simulink model "Session_3"  (R2020b)
settings: Solver=VariableStepAuto  StartTime=0.0  StopTime=inf  RelTol=1e-3
InitFcn:
  | run('Session3.m')
values from neighbouring files (symbols this model uses):
  alpha = 0.2    [Session3.m]
  D1 = randi([0,M-1 ],1,N)    [Session3.m]
  frame = [f22 f11]    [Session3.m]
  header = (-1).^H    [Session3.m]
  hh = numel(H)    [Session3.m]
  L = length(frame)    [Session3.m]
  N = 1e3    (= 1000)    [Session3.m]
  pp = 20    [Session3.m]
  Rs = 1e4    (= 10000)    [Session3.m]
  Span = 10    [Session3.m]
  SPS = 8    [Session3.m]
  stdD = std(D2)    [Session3.m]
undefined symbols (not defined in the file or in its folder): magnitude
libraries: commdigbbndam3 x7, simulink x6, commdigbbndpm3 x6, commfilt2 x2, commchan3 x1, commsink2 x1, dspstat3 x1, dspsrcs4 x1
settings Model: Creator=ali hosseini  LastModifiedBy=ali hosseini

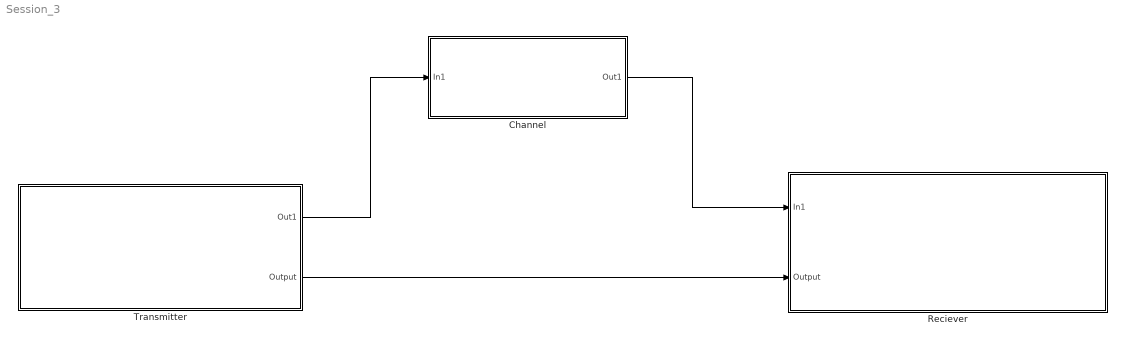
== system Session_3 ==
  Channel : Subsystem
  Reciever : Subsystem
  "Transmitter " : Subsystem
  wires:
  "Transmitter "/2(Output) -> Reciever/2(Output)
  "Transmitter "/1(Out1) -> Channel/1(In1)
  Channel/1(Out1) -> Reciever/1(In1)

== system Session_3/Channel ==
  In1 : Inport
  AWGN Channel : commchan3/AWGN Channel  InputProcessing=Columns as channels (frame based)  seed=67  noiseMode="Signal to noise ratio  (SNR)"  EbNodB=10  EsNodB=10  SNRdB=10000  bitsPerSym=1  Ps=1/SPS  Tsym=1/Rs  variance=1
  Gain : Gain  Gain=0.8
  Out1 : Outport
  wires:
  In1/1 -> AWGN Channel/1
  AWGN Channel/1 -> Gain/1
  Gain/1 -> Out1/1

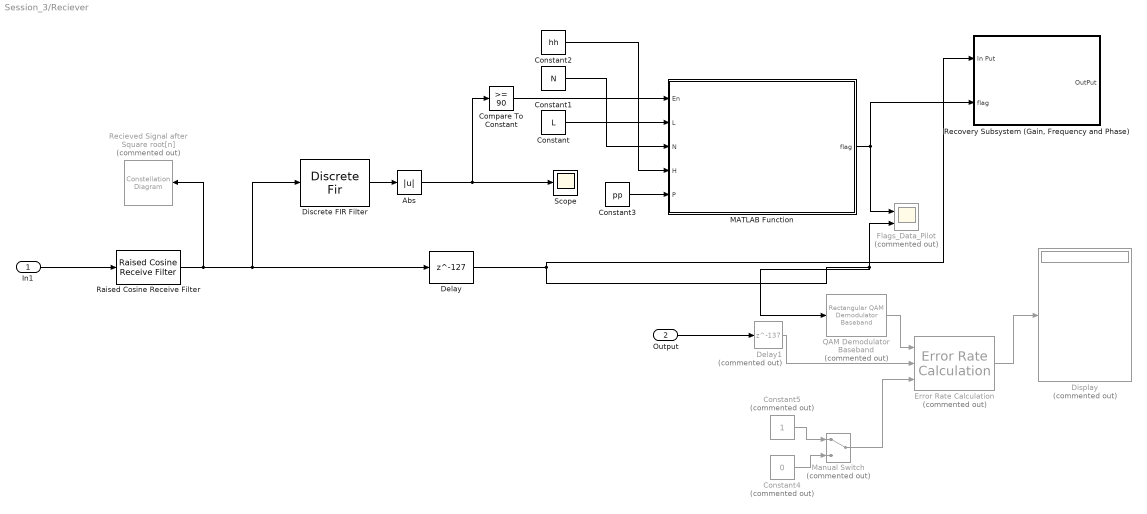
== system Session_3/Reciever ==
  In1 : Inport
  Output : Inport  Port=2
  " QAM Demodulator Baseband" : commdigbbndam3/Rectangular QAM Demodulator Baseband  Commented=on  M=M  OutType=Integer  DecType=Hard decision  VarSource=Dialog  Variance=1  Dec=Gray  Mapping=[0:15]  PowType=Min. distance between symbols  MinDist=2/stdD  AvgPow=1  PeakPow=1  Ph=0  outDtype1=Inherit via internal rule  outDtype2=Inherit via internal rule  derotateFactorWordLen=16  derotateFactorDataTypeStr=Inherit: Same word length as input  derotateFactorLastDataTypeStr=Inherit: Same word length as input  denormFactorWordLen=16  denormFactorDataTypeStr=Inherit: Same word length as input  denormFactorLastDataTypeStr=Inherit: Same word length as input  prodOutWordLen=32  prodOutOverflowMode=Wrap  prodOutRoundingMode=Floor  prodOutOvFlMode=off  prodOutOvFlModeLastStrValue=off  sumWordLen=32
      settings: SourceProductName=Communications Toolbox
  Abs : Abs
  Compare To Constant : simulink/Logic and Bit Operations/Compare To Constant  relop=>=  const=90  OutDataTypeStr=boolean
  Constant : Constant  Value=L  SampleTime=1/Rs
  Constant1 : Constant  Value=N  SampleTime=1/Rs
  Constant2 : Constant  Value=hh  SampleTime=1/Rs
  Constant3 : Constant  Value=pp  SampleTime=1/Rs
  Constant4 : Constant  Commented=on  Value=0
  Constant5 : Constant  Commented=on
  Delay : Delay  DelayLength=127  InputProcessing=Columns as channels (frame based)
  Delay1 : Delay  Commented=on  DelayLength=137
  Discrete FIR Filter : DiscreteFir  Coefficients=fliplr(header)
  Display : Display  Commented=on
  Error Rate Calculation : commsink2/Error Rate Calculation  Commented=on  N=0  st_delay=0  cp_mode=Entire frame  subframe=[]  PMode=Port  WsName=ErrorVec  RsMode2=on  stop=off  numErr=100  maxBits=1e6
  Flags_Data_Pilot : Scope  Commented=on  NumInputPorts=2
  MATLAB Function : MATLAB Function  TreatAsAtomicUnit=on
  Manual Switch : ManualSwitch  Commented=on
  Raised Cosine Receive Filter : commfilt2/Raised Cosine Receive Filter  filtType=Square root  R=alpha  filtSpan=Span  N=SPS  downFactor=SPS  downOffset=0  filterGain=1  InputProcessing=Columns as channels (frame based)  RateOptions=Allow multirate processing  framing=Mute  checkCoeff=off  variableName=rcRxFilt  currentFiltSpan=Span  D=(Span)/2  inputOffset=0  sampMode=Mute  saveAsFlag=0  rateMode=Downsampling  checkGain=Normalized  launchFVT=on  roundingMode=Floor  overflowMode=off  coeffDataTypeStr=Inherit: Same word length as input  coeffMin=[]  coeffMax=[]  coeffLastDataTypeStr=Inherit: Same word length as input  accumDataTypeStr=Inherit: Same as product output  accumLastDataTypeStr=Inherit: Same as product output  outputDataTypeStr=Inherit: Same as accumulator  outputMin=[]  outputMax=[]  outputLastDataTypeStr=Inherit: Same as accumulator
  Recieved Signal after Square root[n] : ConstellationDiagram  Commented=on
  "Recovery Subsystem (Gain, Frequency and Phase)" : Subsystem
  Scope : Scope
  wires:
  In1/1 -> Raised Cosine Receive Filter/1
  Raised Cosine Receive Filter/1 -> Recieved Signal after Square root[n]/1, Delay/1, Discrete FIR Filter/1
  Discrete FIR Filter/1 -> Abs/1
  Abs/1 -> Compare To Constant/1, Scope/1
  Compare To Constant/1 -> MATLAB Function/1(En)
  Constant/1 -> MATLAB Function/2(L)
  Constant1/1 -> MATLAB Function/3(N)
  Constant2/1 -> MATLAB Function/4(H)
  Constant3/1 -> MATLAB Function/5(P)
  MATLAB Function/1(flag) -> Flags_Data_Pilot/1, "Recovery Subsystem (Gain, Frequency and Phase)"/2(flag)
  Delay/1 -> "Recovery Subsystem (Gain, Frequency and Phase)"/1(In Put), " QAM Demodulator Baseband"/1, Flags_Data_Pilot/2
  Constant4/1 -> Manual Switch/2
  Constant5/1 -> Manual Switch/1
  Output/1 -> Delay1/1
  Error Rate Calculation/1 -> Display/1
  Delay1/1 -> Error Rate Calculation/2
  Manual Switch/1 -> Error Rate Calculation/3
  " QAM Demodulator Baseband"/1 -> Error Rate Calculation/1

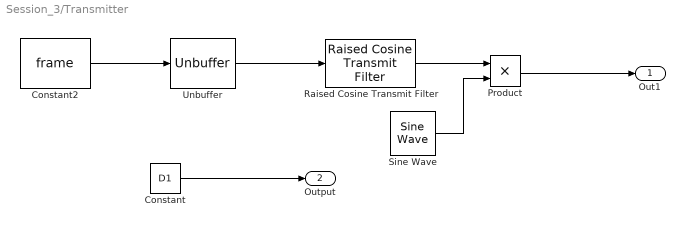
== system Session_3/Transmitter  ==
  Constant : Constant  Value=D1
  Constant2 : Constant  Value=frame  SampleTime=L/Rs  LockScale=on
  Product : Product
  Raised Cosine Transmit Filter : commfilt2/Raised Cosine Transmit Filter  filtType=Square root  R=alpha  filtSpan=Span  N=SPS  filterGain=1  InputProcessing=Columns as channels (frame based)  RateOptions=Allow multirate processing  framing=Mute  checkCoeff=off  variableName=rcTxFilt  checkGain=Normalized  sampMode=Mute  saveAsFlag=0  currentFiltSpan=Span  D=(Span)/2  launchFVT=on  roundingMode=Floor  overflowMode=off  coeffDataTypeStr=Inherit: Same word length as input  coeffMin=[]  coeffMax=[]  coeffLastDataTypeStr=Inherit: Same word length as input  outputDataTypeStr=Inherit: Same as accumulator  outputMin=[]  outputMax=[]  outputLastDataTypeStr=Inherit: Same as accumulator
  Sine Wave : dspsrcs4/Sine Wave  Amplitude=1  Frequency=0.0001*Rs  Phase=3*pi/4  SampleMode=Discrete  OutComplex=Complex  CompMethod=Trigonometric fcn  TableSize=Speed  SampleTime=1/(SPS*Rs)  SamplesPerFrame=1  ResetState=Restart at time zero  OutputFrames=off  dataType=double  wordLen=16  udDataType=sfix(16)  fracBitsMode=Best precision  numFracBits=15  OutDataTypeStr=double  LastOutDataTypeStr=double
  Unbuffer : Unbuffer
  Out1 : Outport
  Output : Outport  Port=2
  wires:
  Unbuffer/1 -> Raised Cosine Transmit Filter/1
  Constant2/1 -> Unbuffer/1
  Raised Cosine Transmit Filter/1 -> Product/1
  Product/1 -> Out1/1
  Constant/1 -> Output/1
  Sine Wave/1 -> Product/2

== system Session_3/Reciever/Recovery Subsystem (Gain, Frequency and Phase) ==
  In Put : Inport
  flag : Inport  Port=2
  AGC : Subsystem
  CFR : Subsystem
  CPR : Subsystem
  OutPut : Outport
  wires:
  flag/1 -> CPR/1(flag), CFR/2(Flags), AGC/2(flag)
  In Put/1 -> AGC/1(In put)
  AGC/1(Out put) -> CFR/1(S)
  CFR/1(Original Signal) -> CPR/2(Original Signal)
  CPR/1(OutPut) -> OutPut/1

== system Session_3/Reciever/Recovery Subsystem (Gain, Frequency and Phase)/AGC ==
  In put : Inport
  flag : Inport  Port=2
  AGC SubSys : Subsystem  TreatAsAtomicUnit=on
  Compare To Constant : simulink/Logic and Bit Operations/Compare To Constant  relop=~=  const=3.0  OutDataTypeStr=boolean
  Delay : Delay  DelayLength=1  InitialCondition=1
  Product : Product
  Out put : Outport
  wires:
  flag/1 -> Compare To Constant/1
  Compare To Constant/1 -> AGC SubSys/Enable
  In put/1 -> Product/1
  AGC SubSys/1(OUt Put) -> Delay/1
  Delay/1 -> Product/2
  Product/1 -> AGC SubSys/1(X), Out put/1

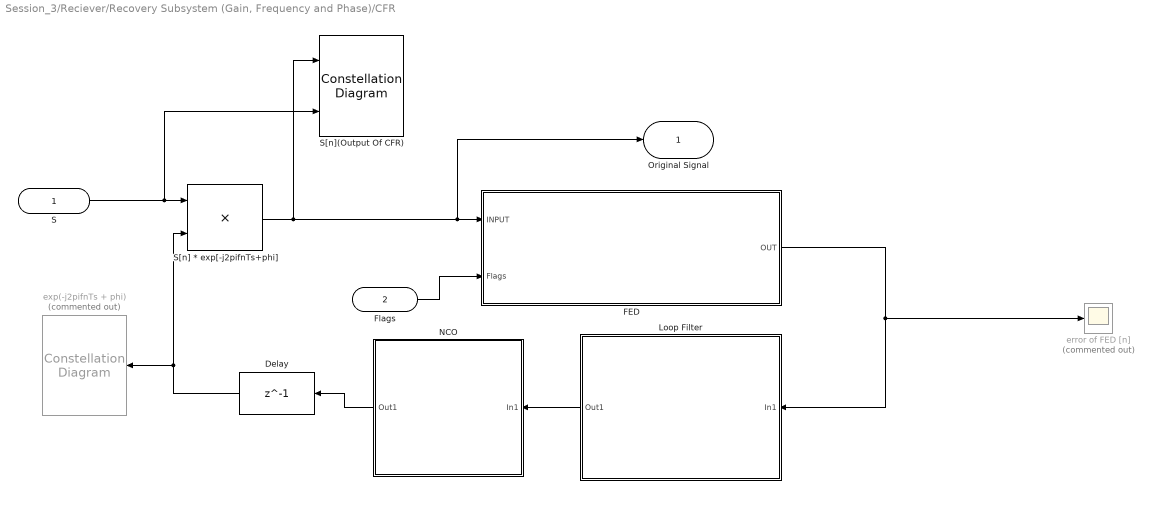
== system Session_3/Reciever/Recovery Subsystem (Gain, Frequency and Phase)/CFR ==
  S : Inport
  Flags : Inport  Port=2
  Delay : Delay  DelayLength=1
  FED : Subsystem
  Loop Filter : Subsystem
  NCO : Subsystem
  S[n] * exp[-j2pifnTs+phi] : Product
  S[n](Output Of CFR) : ConstellationDiagram  NumInputPorts=2
  error of FED [n] : Scope  Commented=on
  exp(-j2pifnTs + phi) : ConstellationDiagram  Commented=on
  Original Signal : Outport
  wires:
  Loop Filter/1(Out1) -> NCO/1(In1)
  NCO/1(Out1) -> Delay/1
  S/1 -> S[n](Output Of CFR)/2, S[n] * exp[-j2pifnTs+phi]/1
  Delay/1 -> exp(-j2pifnTs + phi)/1, S[n] * exp[-j2pifnTs+phi]/2
  S[n] * exp[-j2pifnTs+phi]/1 -> S[n](Output Of CFR)/1, Original Signal/1, FED/1(INPUT)
  Flags/1 -> FED/2(Flags)
  FED/1(OUT) -> Loop Filter/1(In1), error of FED [n]/1

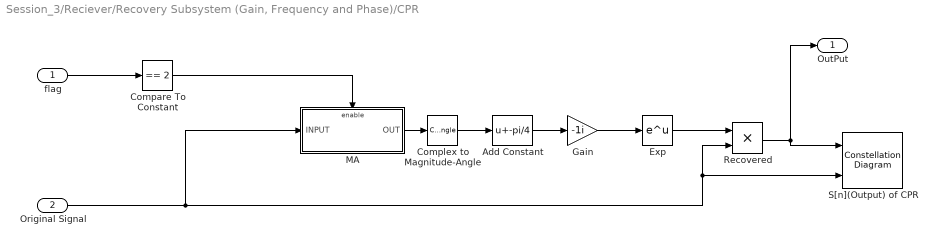
== system Session_3/Reciever/Recovery Subsystem (Gain, Frequency and Phase)/CPR ==
  flag : Inport
  Original Signal : Inport  Port=2
  Add Constant : Bias  Bias=-pi/4
  Compare To Constant : simulink/Logic and Bit Operations/Compare To Constant  relop===  const=2  OutDataTypeStr=boolean
  Complex to Magnitude-Angle : ComplexToMagnitudeAngle  Output=Angle
  Exp : Math  SaturateOnIntegerOverflow=on
  Gain : Gain  Gain=-1i
  MA : Subsystem  TreatAsAtomicUnit=on
  Recovered : Product
  S[n](Output) of CPR : ConstellationDiagram  NumInputPorts=2
  OutPut : Outport
  wires:
  flag/1 -> Compare To Constant/1
  Compare To Constant/1 -> MA/Enable
  Original Signal/1 -> S[n](Output) of CPR/2, Recovered/2, MA/1(INPUT)
  Gain/1 -> Exp/1
  Exp/1 -> Recovered/1
  Recovered/1 -> OutPut/1, S[n](Output) of CPR/1
  MA/1(OUT) -> Complex to Magnitude-Angle/1
  Add Constant/1 -> Gain/1
  Complex to Magnitude-Angle/1 -> Add Constant/1

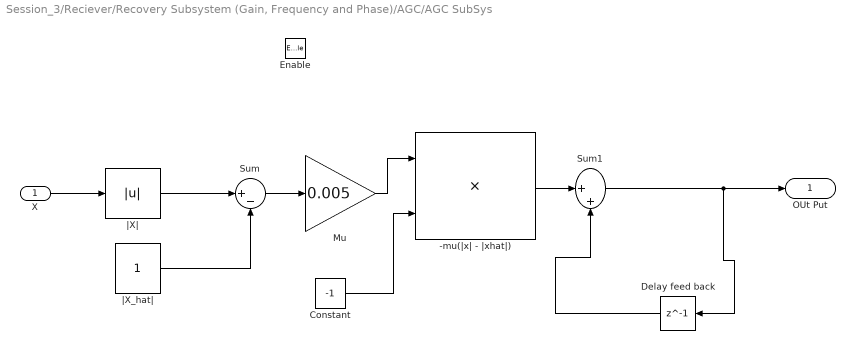
== system Session_3/Reciever/Recovery Subsystem (Gain, Frequency and Phase)/AGC/AGC SubSys ==
  X : Inport
  Enable : EnablePort
  -mu(|x| - |xhat|) : Product
  Constant : Constant  Value=-1
  Delay feed back : Delay  DelayLength=1
  Mu : Gain  Gain=0.005
  Sum : Sum  Inputs=|+-
  Sum1 : Sum  Inputs=|++
  |X_hat| : Constant
  |X| : Abs
  OUt Put : Outport
  wires:
  X/1 -> |X|/1
  |X|/1 -> Sum/1
  |X_hat|/1 -> Sum/2
  Sum/1 -> Mu/1
  Mu/1 -> -mu(|x| - |xhat|)/1
  Constant/1 -> -mu(|x| - |xhat|)/2
  -mu(|x| - |xhat|)/1 -> Sum1/1
  Sum1/1 -> Delay feed back/1, OUt Put/1
  Delay feed back/1 -> Sum1/2

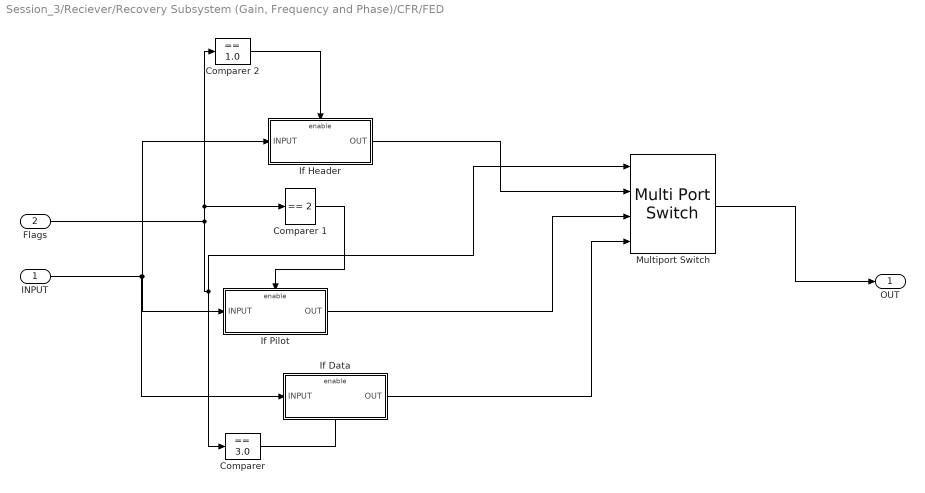
== system Session_3/Reciever/Recovery Subsystem (Gain, Frequency and Phase)/CFR/FED ==
  INPUT : Inport
  Flags : Inport  Port=2
  " If Data" : Subsystem  TreatAsAtomicUnit=on
  "Comparer " : simulink/Logic and Bit Operations/Compare To Constant  relop===  const=3.0  OutDataTypeStr=boolean
  Comparer 1 : simulink/Logic and Bit Operations/Compare To Constant  relop===  const=2  OutDataTypeStr=boolean
  Comparer 2 : simulink/Logic and Bit Operations/Compare To Constant  relop===  const=1.0  OutDataTypeStr=boolean
  If Header : Subsystem  TreatAsAtomicUnit=on
  If Pilot : Subsystem  TreatAsAtomicUnit=on
  Multiport Switch : MultiPortSwitch
  OUT : Outport
  wires:
  INPUT/1 -> " If Data"/1(INPUT), If Pilot/1(INPUT), If Header/1(INPUT)
  Flags/1 -> Multiport Switch/1, "Comparer "/1, Comparer 1/1, Comparer 2/1
  "Comparer "/1 -> " If Data"/Enable
  If Pilot/1(OUT) -> Multiport Switch/3
  Multiport Switch/1 -> OUT/1
  " If Data"/1(OUT) -> Multiport Switch/4
  If Header/1(OUT) -> Multiport Switch/2
  Comparer 1/1 -> If Pilot/Enable
  Comparer 2/1 -> If Header/Enable

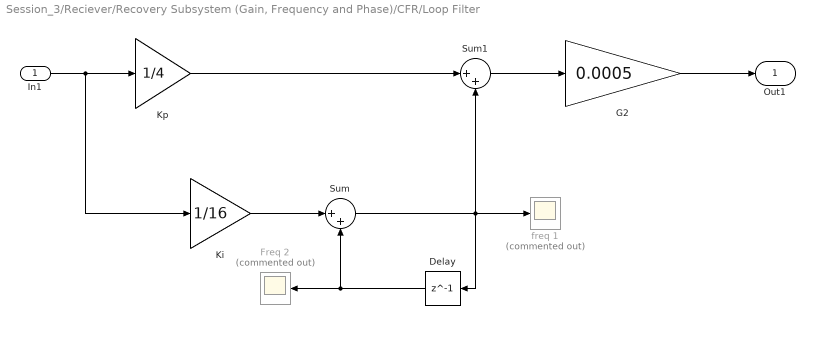
== system Session_3/Reciever/Recovery Subsystem (Gain, Frequency and Phase)/CFR/Loop Filter ==
  In1 : Inport
  Delay : Delay  DelayLength=1
  Freq 2 : Scope  Commented=on
  G2 : Gain  Gain=0.0005
  Ki : Gain  Gain=1/16
  Kp : Gain  Gain=1/4
  Sum : Sum  Inputs=|++
  Sum1 : Sum  Inputs=|++
  freq 1 : Scope  Commented=on
  Out1 : Outport
  wires:
  In1/1 -> Ki/1, Kp/1
  Kp/1 -> Sum1/1
  Ki/1 -> Sum/1
  Delay/1 -> Freq 2/1, Sum/2
  Sum/1 -> freq 1/1, Sum1/2, Delay/1
  Sum1/1 -> G2/1
  G2/1 -> Out1/1

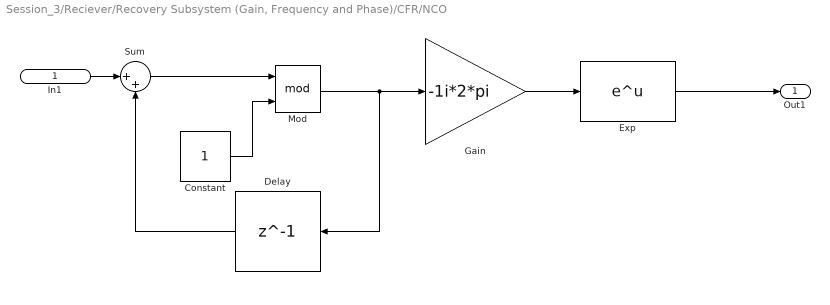
== system Session_3/Reciever/Recovery Subsystem (Gain, Frequency and Phase)/CFR/NCO ==
  In1 : Inport
  Constant : Constant
  Delay : Delay  DelayLength=1
  Exp : Math  SaturateOnIntegerOverflow=on
  Gain : Gain  Gain=-1i*2*pi
  Mod : Math  Operator=mod  SaturateOnIntegerOverflow=on
  Sum : Sum  Inputs=|++
  Out1 : Outport
  wires:
  In1/1 -> Sum/1
  Sum/1 -> Mod/1
  Constant/1 -> Mod/2
  Mod/1 -> Delay/1, Gain/1
  Gain/1 -> Exp/1
  Exp/1 -> Out1/1
  Delay/1 -> Sum/2

== system Session_3/Reciever/Recovery Subsystem (Gain, Frequency and Phase)/CPR/MA ==
  INPUT : Inport
  Enable : EnablePort
  Moving Average : dspstat3/Moving Average  Method=Sliding window  ForgettingFactorPort=off  SpecifyWindowLength=on  WindowLength=24*20  ForgettingFactor=0.9  SimulateUsing=Code generation
  Scope : Scope  NumInputPorts=2
  OUT : Outport
  wires:
  Moving Average/1 -> Scope/1, OUT/1
  INPUT/1 -> Scope/2, Moving Average/1

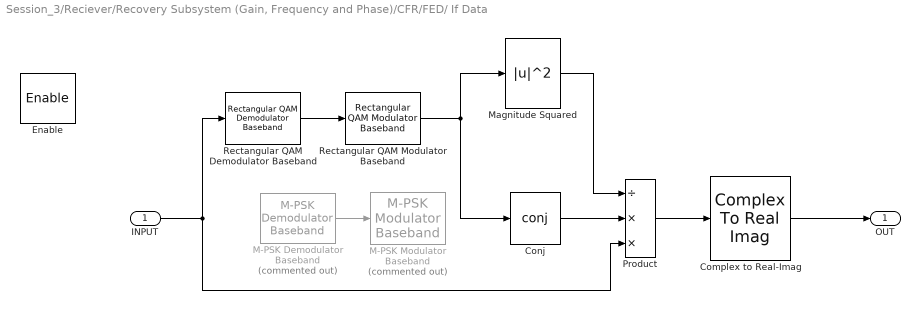
== system Session_3/Reciever/Recovery Subsystem (Gain, Frequency and Phase)/CFR/FED/ If Data ==
  INPUT : Inport
  Enable : EnablePort
  Complex to Real-Imag : ComplexToRealImag  Output=Imag
  Conj : Math  Operator=conj  SaturateOnIntegerOverflow=on
  M-PSK Demodulator Baseband : commdigbbndpm3/M-PSK Demodulator Baseband  Commented=on  M=M  OutType=Integer  DecType=Hard decision  VarSource=Dialog  Variance=1  Dec=Gray  Mapping=[0:7]  Ph=pi/8  outDtype1=Inherit via internal rule  outDtype2=Inherit via internal rule  derotateFactorWordLen=16  derotateFactorDataTypeStr=Inherit: Same word length as input  derotateFactorLastDataTypeStr=Inherit: Same word length as input
      settings: SourceProductName=Communications Toolbox
  M-PSK Modulator Baseband : commdigbbndpm3/M-PSK Modulator Baseband  Commented=on  M=M  InType=Integer  Enc=Gray  Mapping=[0:7]  Ph=pi/8  outDtype=double  outWordLen=16  outUDDataType=sfix(16)  outFracLenMode=Best precision  outFracLen=15  outDataTypeStr=double  outLastDataTypeStr=double
      settings: SourceProductName=Communications Toolbox
  Magnitude Squared : Math  Operator=magnitude^2  SaturateOnIntegerOverflow=on
  Product : Product  Inputs=/**
  Rectangular QAM Demodulator Baseband : commdigbbndam3/Rectangular QAM Demodulator Baseband  M=M  OutType=Integer  DecType=Hard decision  VarSource=Dialog  Variance=1  Dec=Gray  Mapping=[0:15]  PowType=Min. distance between symbols  MinDist=2/stdD  AvgPow=1  PeakPow=1  Ph=0  outDtype1=Inherit via internal rule  outDtype2=Inherit via internal rule  derotateFactorWordLen=16  derotateFactorDataTypeStr=Inherit: Same word length as input  derotateFactorLastDataTypeStr=Inherit: Same word length as input  denormFactorWordLen=16  denormFactorDataTypeStr=Inherit: Same word length as input  denormFactorLastDataTypeStr=Inherit: Same word length as input  prodOutWordLen=32  prodOutOverflowMode=Wrap  prodOutRoundingMode=Floor  prodOutOvFlMode=off  prodOutOvFlModeLastStrValue=off  sumWordLen=32
  Rectangular QAM Modulator Baseband : commdigbbndam3/Rectangular QAM Modulator Baseband  M=M  InType=Integer  Enc=Gray  Mapping=[0:15]  PowType=Min. distance between symbols  MinDist=2/stdD  AvgPow=1  PeakPow=1  Ph=0  outDtype=double  outWordLen=16  outUDDataType=sfix(16)  outFracLenMode=Best precision  outFracLen=15  outDataTypeStr=double  outLastDataTypeStr=double
  OUT : Outport
  wires:
  Complex to Real-Imag/1 -> OUT/1
  Product/1 -> Complex to Real-Imag/1
  INPUT/1 -> Rectangular QAM Demodulator Baseband/1, Product/3
  Conj/1 -> Product/2
  M-PSK Demodulator Baseband/1 -> M-PSK Modulator Baseband/1
  Magnitude Squared/1 -> Product/1
  Rectangular QAM Modulator Baseband/1 -> Magnitude Squared/1, Conj/1
  Rectangular QAM Demodulator Baseband/1 -> Rectangular QAM Modulator Baseband/1

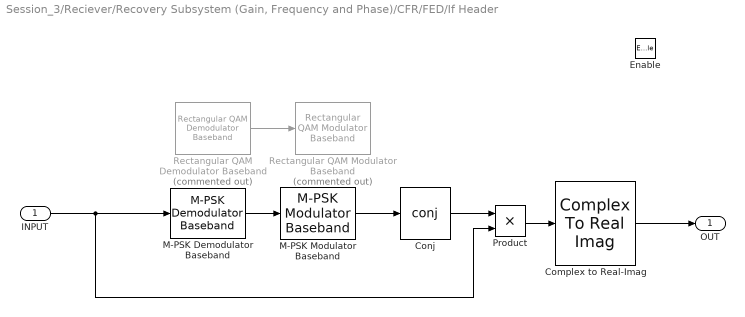
== system Session_3/Reciever/Recovery Subsystem (Gain, Frequency and Phase)/CFR/FED/If Header ==
  INPUT : Inport
  Enable : EnablePort
  Complex to Real-Imag : ComplexToRealImag  Output=Imag
  Conj : Math  Operator=conj  SaturateOnIntegerOverflow=on
  M-PSK Demodulator Baseband : commdigbbndpm3/M-PSK Demodulator Baseband  M=2  OutType=Integer  DecType=Hard decision  VarSource=Dialog  Variance=1  Dec=Gray  Mapping=[0:7]  Ph=0  outDtype1=Inherit via internal rule  outDtype2=Inherit via internal rule  derotateFactorWordLen=16  derotateFactorDataTypeStr=Inherit: Same word length as input  derotateFactorLastDataTypeStr=Inherit: Same word length as input
      settings: SourceProductName=Communications Toolbox
  M-PSK Modulator Baseband : commdigbbndpm3/M-PSK Modulator Baseband  M=2  InType=Integer  Enc=Gray  Mapping=[0:7]  Ph=0  outDtype=double  outWordLen=16  outUDDataType=sfix(16)  outFracLenMode=Best precision  outFracLen=15  outDataTypeStr=double  outLastDataTypeStr=double
      settings: SourceProductName=Communications Toolbox
  Product : Product
  Rectangular QAM Demodulator Baseband : commdigbbndam3/Rectangular QAM Demodulator Baseband  Commented=on  M=M  OutType=Integer  DecType=Hard decision  VarSource=Dialog  Variance=1  Dec=Gray  Mapping=[0:15]  PowType=Min. distance between symbols  MinDist=2  AvgPow=1  PeakPow=1  Ph=0  outDtype1=Inherit via internal rule  outDtype2=Inherit via internal rule  derotateFactorWordLen=16  derotateFactorDataTypeStr=Inherit: Same word length as input  derotateFactorLastDataTypeStr=Inherit: Same word length as input  denormFactorWordLen=16  denormFactorDataTypeStr=Inherit: Same word length as input  denormFactorLastDataTypeStr=Inherit: Same word length as input  prodOutWordLen=32  prodOutOverflowMode=Wrap  prodOutRoundingMode=Floor  prodOutOvFlMode=off  prodOutOvFlModeLastStrValue=off  sumWordLen=32
      settings: SourceProductName=Communications Toolbox
  Rectangular QAM Modulator Baseband : commdigbbndam3/Rectangular QAM Modulator Baseband  Commented=on  M=M  InType=Integer  Enc=Gray  Mapping=[0:15]  PowType=Min. distance between symbols  MinDist=2  AvgPow=1  PeakPow=1  Ph=0  outDtype=double  outWordLen=16  outUDDataType=sfix(16)  outFracLenMode=Best precision  outFracLen=15  outDataTypeStr=double  outLastDataTypeStr=double
      settings: SourceProductName=Communications Toolbox
  OUT : Outport
  wires:
  INPUT/1 -> M-PSK Demodulator Baseband/1, Product/2
  Conj/1 -> Product/1
  Product/1 -> Complex to Real-Imag/1
  Complex to Real-Imag/1 -> OUT/1
  M-PSK Demodulator Baseband/1 -> M-PSK Modulator Baseband/1
  Rectangular QAM Demodulator Baseband/1 -> Rectangular QAM Modulator Baseband/1
  M-PSK Modulator Baseband/1 -> Conj/1

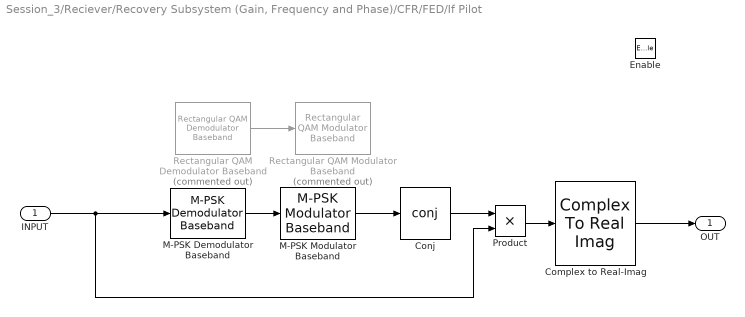
== system Session_3/Reciever/Recovery Subsystem (Gain, Frequency and Phase)/CFR/FED/If Pilot ==
  INPUT : Inport
  Enable : EnablePort
  Complex to Real-Imag : ComplexToRealImag  Output=Imag
  Conj : Math  Operator=conj  SaturateOnIntegerOverflow=on
  M-PSK Demodulator Baseband : commdigbbndpm3/M-PSK Demodulator Baseband  M=4  OutType=Integer  DecType=Hard decision  VarSource=Dialog  Variance=1  Dec=Gray  Mapping=[0:7]  Ph=pi/4  outDtype1=Inherit via internal rule  outDtype2=Inherit via internal rule  derotateFactorWordLen=16  derotateFactorDataTypeStr=Inherit: Same word length as input  derotateFactorLastDataTypeStr=Inherit: Same word length as input
      settings: SourceProductName=Communications Toolbox
  M-PSK Modulator Baseband : commdigbbndpm3/M-PSK Modulator Baseband  M=4  InType=Integer  Enc=Gray  Mapping=[0:7]  Ph=pi/4  outDtype=double  outWordLen=16  outUDDataType=sfix(16)  outFracLenMode=Best precision  outFracLen=15  outDataTypeStr=double  outLastDataTypeStr=double
      settings: SourceProductName=Communications Toolbox
  Product : Product
  Rectangular QAM Demodulator Baseband : commdigbbndam3/Rectangular QAM Demodulator Baseband  Commented=on  M=M  OutType=Integer  DecType=Hard decision  VarSource=Dialog  Variance=1  Dec=Gray  Mapping=[0:15]  PowType=Min. distance between symbols  MinDist=2  AvgPow=1  PeakPow=1  Ph=0  outDtype1=Inherit via internal rule  outDtype2=Inherit via internal rule  derotateFactorWordLen=16  derotateFactorDataTypeStr=Inherit: Same word length as input  derotateFactorLastDataTypeStr=Inherit: Same word length as input  denormFactorWordLen=16  denormFactorDataTypeStr=Inherit: Same word length as input  denormFactorLastDataTypeStr=Inherit: Same word length as input  prodOutWordLen=32  prodOutOverflowMode=Wrap  prodOutRoundingMode=Floor  prodOutOvFlMode=off  prodOutOvFlModeLastStrValue=off  sumWordLen=32
      settings: SourceProductName=Communications Toolbox
  Rectangular QAM Modulator Baseband : commdigbbndam3/Rectangular QAM Modulator Baseband  Commented=on  M=M  InType=Integer  Enc=Gray  Mapping=[0:15]  PowType=Min. distance between symbols  MinDist=2  AvgPow=1  PeakPow=1  Ph=0  outDtype=double  outWordLen=16  outUDDataType=sfix(16)  outFracLenMode=Best precision  outFracLen=15  outDataTypeStr=double  outLastDataTypeStr=double
      settings: SourceProductName=Communications Toolbox
  OUT : Outport
  wires:
  INPUT/1 -> M-PSK Demodulator Baseband/1, Product/2
  Conj/1 -> Product/1
  Product/1 -> Complex to Real-Imag/1
  Complex to Real-Imag/1 -> OUT/1
  M-PSK Demodulator Baseband/1 -> M-PSK Modulator Baseband/1
  Rectangular QAM Demodulator Baseband/1 -> Rectangular QAM Modulator Baseband/1
  M-PSK Modulator Baseband/1 -> Conj/1

== matlab function Session_3/Reciever/MATLAB Function ==
  data: En input; flag output; L input; N input; H input; P input
function flag = flagDet(En,L,N,H,P)
    persistent n ;
    if isempty(n)
        n = 0;
    end
    
    flag = 3; %Data 
    if n < H
        flag = 1 ; %header
    elseif  ( n >= H + N && n < H + N +  P) || ( n >= H + 2*N + P && n < 2*P + 2*N + H)
        flag = 2; %Pilot
    end
    
    if En
        n = 0 ;
    end
    n = mod(n + 1 , L);
end
